simulink model "Ass3Q2_1"  (R2018b)
settings: Solver=VariableStepAuto  StartTime=0.0  StopTime=10.0  RelTol=1e-3
values from neighbouring files (symbols this model uses):
  K = K(1,:)    [Adaptive3.m]
  l = 50/1.5    (= 33.3333333333)    [Adaptive3.m]
undefined symbols (not defined in the file or in its folder): ss_mo, ss_pl
settings Model: Creator=bigfoot  LastModifiedBy=bigfoot

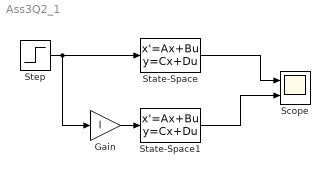
== system Ass3Q2_1 ==
  Gain : Gain  Gain=l
  Scope : Scope  NumInputPorts=2
  State-Space : StateSpace  A=ss_mo.a  B=ss_mo.b  C=ss_mo.c  D=ss_mo.d  InitialCondition=0
  State-Space1 : StateSpace  A=ss_pl.a-ss_pl.b*K  B=ss_pl.b  C=ss_pl.c  D=[0]  InitialCondition=0
  Step : Step  SampleTime=0
  wires:
  State-Space1/1 -> Scope/2
  State-Space/1 -> Scope/1
  Step/1 -> Gain/1, State-Space/1
  Gain/1 -> State-Space1/1
